simulink model "x20240109_HVDCMMCInterconnection"  (R2023b)
settings: Solver=FixedStepDiscrete  StartTime=0.0  StopTime=2  FixedStep=Ts_Power  RelTol=1e-4  EnableMultiTasking=on
PreLoadFcn:
  | HVDCMMCInterconnectionParam
StartFcn:
  | tic
StopFcn:
  | toc
values from neighbouring files (symbols this model uses):
  C_PM = 1.758e-3    (= 0.001758)    [HVDCMMCInterconnectionParam.m]
  Cg = 50e-9    (= 5e-08)    [HVDCMMCInterconnectionParam.m]
  D_R = 0.001    [HVDCMMCInterconnectionParam.m]
  D_Rs = 1e8    (= 100000000)    [HVDCMMCInterconnectionParam.m]
  D_Vf = 0    [HVDCMMCInterconnectionParam.m]
  Fnom = 50    [HVDCMMCInterconnectionParam.m]
  HRM = 2    [HVDCMMCInterconnectionParam.m]
  Ki_Ireg = 6    [HVDCMMCInterconnectionParam.m]
  Ki_Preg = 1.0    (= 1)    [HVDCMMCInterconnectionParam.m]
  Ki_Qreg = 1.0    (= 1)    [HVDCMMCInterconnectionParam.m]
  Ki_VDCreg = 100    [HVDCMMCInterconnectionParam.m]
  Kp_Ireg = 0.6    [HVDCMMCInterconnectionParam.m]
  Kp_Preg = 0.5/3    (= 0.166666666667)    [HVDCMMCInterconnectionParam.m]
  Kp_Qreg = 0.5/3    (= 0.166666666667)    [HVDCMMCInterconnectionParam.m]
  Kp_VDCreg = 4    [HVDCMMCInterconnectionParam.m]
  L_cable = 15e-3    (= 0.015)    [HVDCMMCInterconnectionParam.m]
  Larm = Larm_pu*(Zb_ac/(2*pi*Fnom))    [HVDCMMCInterconnectionParam.m]
  Lff = Larm_pu/2    (= 0.075)    [HVDCMMCInterconnectionParam.m]
  Limits_Ireg = [ 2.0  -2.0]    [HVDCMMCInterconnectionParam.m]
  Limits_Preg = [ 1.2, 0.8 ]    [HVDCMMCInterconnectionParam.m]
  Limits_Qreg = [ 0.25, -0.25 ]    [HVDCMMCInterconnectionParam.m]
  Limits_VDCreg = [ 2.0  -2.0]    [HVDCMMCInterconnectionParam.m]
  Lxfo = 0.12    [HVDCMMCInterconnectionParam.m]
  Nb_PM = 36    [HVDCMMCInterconnectionParam.m]
  Pnom = 1000e6    (= 1000000000)    [HVDCMMCInterconnectionParam.m]
  R_cable = 0.5    [HVDCMMCInterconnectionParam.m]
  R_startup = 400    [HVDCMMCInterconnectionParam.m]
  Rarm = Rarm_pu*Zb_ac    [HVDCMMCInterconnectionParam.m]
  Rff = Rarm_pu/2    (= 0.00075)    [HVDCMMCInterconnectionParam.m]
  Rg = 100    [HVDCMMCInterconnectionParam.m]
  Rxfo = 0.003    [HVDCMMCInterconnectionParam.m]
  Slope_Pref = 0.5    [HVDCMMCInterconnectionParam.m]
  Slope_Qref = 0.5    [HVDCMMCInterconnectionParam.m]
  Slope_Vdc_ref = Vnom_dc/5    (= 128000)    [HVDCMMCInterconnectionParam.m]
  Tbrk1_On = 0.1    [HVDCMMCInterconnectionParam.m]
  Tbrk2_On = 1.0    (= 1)    [HVDCMMCInterconnectionParam.m]
  Tdeblock = 1.5    [HVDCMMCInterconnectionParam.m]
  Tfault = 9999    [HVDCMMCInterconnectionParam.m]
  Ton_Converter2 = 4    [HVDCMMCInterconnectionParam.m]
  Ton_PQreg = 4    [HVDCMMCInterconnectionParam.m]
  Ton_VDCreg = 1.5    [HVDCMMCInterconnectionParam.m]
  Ts = Ts_Control    (= 4e-05)    [HVDCMMCInterconnectionParam.m]
  Ts_Control = 40e-6    (= 4e-05)    [HVDCMMCInterconnectionParam.m]
  Ts_Power = 20e-6    (= 2e-05)    [HVDCMMCInterconnectionParam.m]
  Vb_ac = sqrt(2/3)*Vnom_sec    [HVDCMMCInterconnectionParam.m]
  Vb_dc = Vnom_dc    (= 640000)    [HVDCMMCInterconnectionParam.m]
  Vc0_PM = 0    [HVDCMMCInterconnectionParam.m]
  Vnom_dc = 640e3    (= 640000)    [HVDCMMCInterconnectionParam.m]
  Vnom_prim = 400e3    (= 400000)    [HVDCMMCInterconnectionParam.m]
  Vnom_sec = 333e3    (= 333000)    [HVDCMMCInterconnectionParam.m]
  w = 2*pi*Fnom    (= 314.159265359)    [HVDCMMCInterconnectionParam.m]
undefined symbols (not defined in the file or in its folder): DiscIntNeverNeededParam, gcbh, Pcc, S, sps_AC, sps_ACDC2, sps_rtmsupport
libraries: simulink x48, spsControlledVoltageSourceLib x30, spsCurrentMeasurementLib x30, MMC_Lib x30, spsDiodeLib x20, spsSeriesRLCBranchLib x14, powerlib_extras x12, spsVoltageMeasurementLib x12, spsSecondOrderFilterLib x8, spsabctodq0Lib x8, spsGroundLib x7, spsMeanLib x4
(part 2 of 9)

== system x20240109_HVDCMMCInterconnection/3ph SM11 ==
  Uref_An : Inport
  An_Ipos : Inport  Port=2
  An_Icap : Inport  Port=3
  Demux : Demux  Outputs=2
  Demux2 : Demux  Outputs=2
  Discrete-Time Integrator1 : DiscreteIntegrator  IntegratorMethod=Integration: Trapezoidal  gainval=1  SampleTime=Ts_Power  UpperSaturationLimit=5000  LowerSaturationLimit=500  ICPrevOutput=DiscIntNeverNeededParam  ICPrevScaledInput=DiscIntNeverNeededParam
  Gain1 : Gain  Gain=Nb_PM
  Gain4 : Gain  Gain=1/(C_PM*Nb_PM)
  Gain5 : Gain  Gain=2
  Mux1 : Mux  Inputs=2
  Mux2 : Mux  Inputs=2
  Product3 : Product
  Product4 : Product
  Product7 : Product
  Sum3 : Sum  Inputs=1  InputSameDT=on  SaturateOnIntegerOverflow=on  OutDataTypeStr=Inherit: Same as first input
  Sum4 : Sum  Inputs=+-  InputSameDT=on  SaturateOnIntegerOverflow=on  OutDataTypeStr=Inherit: Same as first input
  Unit Delay5 : UnitDelay  SampleTime=Ts_Power  HasFrameUpgradeWarning=on
  Unit Delay6 : UnitDelay  SampleTime=Ts_Power  HasFrameUpgradeWarning=on
  Unit Delay7 : UnitDelay  SampleTime=Ts_Power  HasFrameUpgradeWarning=on
  An_Vbl : Outport
  An_Vin : Outport  Port=2
  wires:
  Gain5/1 -> Sum4/1
  Gain1/1 -> Demux2/1, Product3/1
  Mux2/1 -> Demux/1
  Demux/1 -> An_Vin/1
  Uref_An/1 -> Gain1/1
  Gain4/1 -> Discrete-Time Integrator1/1
  Mux1/1 -> Unit Delay7/1
  Demux2/2 -> Product7/1
  Unit Delay6/1 -> Gain5/1, Unit Delay5/1
  An_Icap/1 -> Mux1/2
  Demux2/1 -> Product4/1
  Discrete-Time Integrator1/1 -> Unit Delay6/1
  Sum4/1 -> Product7/2, Product4/2  "Vc"
  Unit Delay5/1 -> Sum4/2
  Sum3/1 -> Gain4/1
  Product3/1 -> Sum3/1
  Product4/1 -> Mux2/1  "Vin"
  Demux/2 -> An_Vbl/1
  Product7/1 -> Mux2/2  "Vbl"
  Unit Delay7/1 -> Product3/2
  An_Ipos/1 -> Mux1/1

== system x20240109_HVDCMMCInterconnection/3ph SM12 ==
  Uref_An : Inport
  An_Ipos : Inport  Port=2
  An_Icap : Inport  Port=3
  Demux : Demux  Outputs=2
  Demux2 : Demux  Outputs=2
  Discrete-Time Integrator1 : DiscreteIntegrator  IntegratorMethod=Integration: Trapezoidal  gainval=1  SampleTime=Ts_Power  UpperSaturationLimit=5000  LowerSaturationLimit=500  ICPrevOutput=DiscIntNeverNeededParam  ICPrevScaledInput=DiscIntNeverNeededParam
  Gain1 : Gain  Gain=Nb_PM
  Gain4 : Gain  Gain=1/(C_PM*Nb_PM)
  Gain5 : Gain  Gain=2
  Mux1 : Mux  Inputs=2
  Mux2 : Mux  Inputs=2
  Product3 : Product
  Product4 : Product
  Product7 : Product
  Sum3 : Sum  Inputs=1  InputSameDT=on  SaturateOnIntegerOverflow=on  OutDataTypeStr=Inherit: Same as first input
  Sum4 : Sum  Inputs=+-  InputSameDT=on  SaturateOnIntegerOverflow=on  OutDataTypeStr=Inherit: Same as first input
  Unit Delay5 : UnitDelay  SampleTime=Ts_Power  HasFrameUpgradeWarning=on
  Unit Delay6 : UnitDelay  SampleTime=Ts_Power  HasFrameUpgradeWarning=on
  Unit Delay7 : UnitDelay  SampleTime=Ts_Power  HasFrameUpgradeWarning=on
  An_Vbl : Outport
  An_Vin : Outport  Port=2
  wires:
  Gain5/1 -> Sum4/1
  Gain1/1 -> Demux2/1, Product3/1
  Mux2/1 -> Demux/1
  Demux/1 -> An_Vin/1
  Uref_An/1 -> Gain1/1
  Gain4/1 -> Discrete-Time Integrator1/1
  Mux1/1 -> Unit Delay7/1
  Demux2/2 -> Product7/1
  Unit Delay6/1 -> Gain5/1, Unit Delay5/1
  An_Icap/1 -> Mux1/2
  Demux2/1 -> Product4/1
  Discrete-Time Integrator1/1 -> Unit Delay6/1
  Sum4/1 -> Product7/2, Product4/2  "Vc"
  Unit Delay5/1 -> Sum4/2
  Sum3/1 -> Gain4/1
  Product3/1 -> Sum3/1
  Product4/1 -> Mux2/1  "Vin"
  Demux/2 -> An_Vbl/1
  Product7/1 -> Mux2/2  "Vbl"
  Unit Delay7/1 -> Product3/2
  An_Ipos/1 -> Mux1/1

== system x20240109_HVDCMMCInterconnection/3ph SM13 ==
  Uref_An : Inport
  An_Ipos : Inport  Port=2
  An_Icap : Inport  Port=3
  Demux : Demux  Outputs=2
  Demux2 : Demux  Outputs=2
  Discrete-Time Integrator1 : DiscreteIntegrator  IntegratorMethod=Integration: Trapezoidal  gainval=1  SampleTime=Ts_Power  UpperSaturationLimit=5000  LowerSaturationLimit=500  ICPrevOutput=DiscIntNeverNeededParam  ICPrevScaledInput=DiscIntNeverNeededParam
  Gain1 : Gain  Gain=Nb_PM
  Gain4 : Gain  Gain=1/(C_PM*Nb_PM)
  Gain5 : Gain  Gain=2
  Mux1 : Mux  Inputs=2
  Mux2 : Mux  Inputs=2
  Product3 : Product
  Product4 : Product
  Product7 : Product
  Sum3 : Sum  Inputs=1  InputSameDT=on  SaturateOnIntegerOverflow=on  OutDataTypeStr=Inherit: Same as first input
  Sum4 : Sum  Inputs=+-  InputSameDT=on  SaturateOnIntegerOverflow=on  OutDataTypeStr=Inherit: Same as first input
  Unit Delay5 : UnitDelay  SampleTime=Ts_Power  HasFrameUpgradeWarning=on
  Unit Delay6 : UnitDelay  SampleTime=Ts_Power  HasFrameUpgradeWarning=on
  Unit Delay7 : UnitDelay  SampleTime=Ts_Power  HasFrameUpgradeWarning=on
  An_Vbl : Outport
  An_Vin : Outport  Port=2
  wires:
  Gain5/1 -> Sum4/1
  Gain1/1 -> Demux2/1, Product3/1
  Mux2/1 -> Demux/1
  Demux/1 -> An_Vin/1
  Uref_An/1 -> Gain1/1
  Gain4/1 -> Discrete-Time Integrator1/1
  Mux1/1 -> Unit Delay7/1
  Demux2/2 -> Product7/1
  Unit Delay6/1 -> Gain5/1, Unit Delay5/1
  An_Icap/1 -> Mux1/2
  Demux2/1 -> Product4/1
  Discrete-Time Integrator1/1 -> Unit Delay6/1
  Sum4/1 -> Product7/2, Product4/2  "Vc"
  Unit Delay5/1 -> Sum4/2
  Sum3/1 -> Gain4/1
  Product3/1 -> Sum3/1
  Product4/1 -> Mux2/1  "Vin"
  Demux/2 -> An_Vbl/1
  Product7/1 -> Mux2/2  "Vbl"
  Unit Delay7/1 -> Product3/2
  An_Ipos/1 -> Mux1/1

== system x20240109_HVDCMMCInterconnection/3ph SM14 ==
  Uref_An : Inport
  An_Ipos : Inport  Port=2
  An_Icap : Inport  Port=3
  Demux : Demux  Outputs=2
  Demux2 : Demux  Outputs=2
  Discrete-Time Integrator1 : DiscreteIntegrator  IntegratorMethod=Integration: Trapezoidal  gainval=1  SampleTime=Ts_Power  UpperSaturationLimit=5000  LowerSaturationLimit=500  ICPrevOutput=DiscIntNeverNeededParam  ICPrevScaledInput=DiscIntNeverNeededParam
  Gain1 : Gain  Gain=Nb_PM
  Gain4 : Gain  Gain=1/(C_PM*Nb_PM)
  Gain5 : Gain  Gain=2
  Mux1 : Mux  Inputs=2
  Mux2 : Mux  Inputs=2
  Product3 : Product
  Product4 : Product
  Product7 : Product
  Sum3 : Sum  Inputs=1  InputSameDT=on  SaturateOnIntegerOverflow=on  OutDataTypeStr=Inherit: Same as first input
  Sum4 : Sum  Inputs=+-  InputSameDT=on  SaturateOnIntegerOverflow=on  OutDataTypeStr=Inherit: Same as first input
  Unit Delay5 : UnitDelay  SampleTime=Ts_Power  HasFrameUpgradeWarning=on
  Unit Delay6 : UnitDelay  SampleTime=Ts_Power  HasFrameUpgradeWarning=on
  Unit Delay7 : UnitDelay  SampleTime=Ts_Power  HasFrameUpgradeWarning=on
  An_Vbl : Outport
  An_Vin : Outport  Port=2
  wires:
  Gain5/1 -> Sum4/1
  Gain1/1 -> Demux2/1, Product3/1
  Mux2/1 -> Demux/1
  Demux/1 -> An_Vin/1
  Uref_An/1 -> Gain1/1
  Gain4/1 -> Discrete-Time Integrator1/1
  Mux1/1 -> Unit Delay7/1
  Demux2/2 -> Product7/1
  Unit Delay6/1 -> Gain5/1, Unit Delay5/1
  An_Icap/1 -> Mux1/2
  Demux2/1 -> Product4/1
  Discrete-Time Integrator1/1 -> Unit Delay6/1
  Sum4/1 -> Product7/2, Product4/2  "Vc"
  Unit Delay5/1 -> Sum4/2
  Sum3/1 -> Gain4/1
  Product3/1 -> Sum3/1
  Product4/1 -> Mux2/1  "Vin"
  Demux/2 -> An_Vbl/1
  Product7/1 -> Mux2/2  "Vbl"
  Unit Delay7/1 -> Product3/2
  An_Ipos/1 -> Mux1/1

== system x20240109_HVDCMMCInterconnection/3ph SM2 ==
  Uref_Ap : Inport
  Ap_Ipos : Inport  Port=2
  Ap_Icap : Inport  Port=3
  Demux1 : Demux  Outputs=2
  Demux3 : Demux  Outputs=2
  Discrete-Time Integrator2 : DiscreteIntegrator  IntegratorMethod=Integration: Trapezoidal  gainval=1  SampleTime=Ts_Power  UpperSaturationLimit=5000  LowerSaturationLimit=500  ICPrevOutput=DiscIntNeverNeededParam  ICPrevScaledInput=DiscIntNeverNeededParam
  Gain2 : Gain  Gain=Nb_PM
  Gain3 : Gain  Gain=1/(C_PM*Nb_PM)
  Gain6 : Gain  Gain=2
  Mux3 : Mux  Inputs=2
  Mux4 : Mux  Inputs=2
  Product1 : Product
  Product2 : Product
  Product5 : Product
  Sum1 : Sum  Inputs=1  InputSameDT=on  SaturateOnIntegerOverflow=on  OutDataTypeStr=Inherit: Same as first input
  Sum2 : Sum  Inputs=+-  InputSameDT=on  SaturateOnIntegerOverflow=on  OutDataTypeStr=Inherit: Same as first input
  Unit Delay1 : UnitDelay  SampleTime=Ts_Power  HasFrameUpgradeWarning=on
  Unit Delay2 : UnitDelay  SampleTime=Ts_Power  HasFrameUpgradeWarning=on
  Unit Delay3 : UnitDelay  SampleTime=Ts_Power  HasFrameUpgradeWarning=on
  Ap_Vbl : Outport
  Ap_Vin : Outport  Port=2
  wires:
  Demux1/2 -> Ap_Vbl/1
  Ap_Ipos/1 -> Mux3/1
  Unit Delay3/1 -> Product1/2
  Product1/1 -> Sum1/1
  Sum1/1 -> Gain3/1
  Unit Delay1/1 -> Sum2/2
  Sum2/1 -> Product5/2, Product2/2  "Vc"
  Uref_Ap/1 -> Gain2/1
  Unit Delay2/1 -> Gain6/1, Unit Delay1/1
  Mux3/1 -> Unit Delay3/1
  Demux3/2 -> Product5/1
  Gain3/1 -> Discrete-Time Integrator2/1
  Gain2/1 -> Demux3/1, Product1/1
  Demux3/1 -> Product2/1
  Demux1/1 -> Ap_Vin/1
  Mux4/1 -> Demux1/1
  Product2/1 -> Mux4/1  "Vin"
  Discrete-Time Integrator2/1 -> Unit Delay2/1
  Ap_Icap/1 -> Mux3/2
  Gain6/1 -> Sum2/1
  Product5/1 -> Mux4/2  "Vbl"

== system x20240109_HVDCMMCInterconnection/3ph SM9 ==
  Uref_An : Inport
  An_Ipos : Inport  Port=2
  An_Icap : Inport  Port=3
  Demux : Demux  Outputs=2
  Demux2 : Demux  Outputs=2
  Discrete-Time Integrator1 : DiscreteIntegrator  IntegratorMethod=Integration: Trapezoidal  gainval=1  SampleTime=Ts_Power  UpperSaturationLimit=5000  LowerSaturationLimit=500  ICPrevOutput=DiscIntNeverNeededParam  ICPrevScaledInput=DiscIntNeverNeededParam
  Gain1 : Gain  Gain=Nb_PM
  Gain4 : Gain  Gain=1/(C_PM*Nb_PM)
  Gain5 : Gain  Gain=2
  Mux1 : Mux  Inputs=2
  Mux2 : Mux  Inputs=2
  Product3 : Product
  Product4 : Product
  Product7 : Product
  Sum3 : Sum  Inputs=1  InputSameDT=on  SaturateOnIntegerOverflow=on  OutDataTypeStr=Inherit: Same as first input
  Sum4 : Sum  Inputs=+-  InputSameDT=on  SaturateOnIntegerOverflow=on  OutDataTypeStr=Inherit: Same as first input
  Unit Delay5 : UnitDelay  SampleTime=Ts_Power  HasFrameUpgradeWarning=on
  Unit Delay6 : UnitDelay  SampleTime=Ts_Power  HasFrameUpgradeWarning=on
  Unit Delay7 : UnitDelay  SampleTime=Ts_Power  HasFrameUpgradeWarning=on
  An_Vbl : Outport
  An_Vin : Outport  Port=2
  wires:
  Gain5/1 -> Sum4/1
  Gain1/1 -> Demux2/1, Product3/1
  Mux2/1 -> Demux/1
  Demux/1 -> An_Vin/1
  Uref_An/1 -> Gain1/1
  Gain4/1 -> Discrete-Time Integrator1/1
  Mux1/1 -> Unit Delay7/1
  Demux2/2 -> Product7/1
  Unit Delay6/1 -> Gain5/1, Unit Delay5/1
  An_Icap/1 -> Mux1/2
  Demux2/1 -> Product4/1
  Discrete-Time Integrator1/1 -> Unit Delay6/1
  Sum4/1 -> Product7/2, Product4/2  "Vc"
  Unit Delay5/1 -> Sum4/2
  Sum3/1 -> Gain4/1
  Product3/1 -> Sum3/1
  Product4/1 -> Mux2/1  "Vin"
  Demux/2 -> An_Vbl/1
  Product7/1 -> Mux2/2  "Vbl"
  Unit Delay7/1 -> Product3/2
  An_Ipos/1 -> Mux1/1

== system x20240109_HVDCMMCInterconnection/Control ==
  PQreg_ON : Inport
  Vdc_ref : Inport  Port=2
  Qref : Inport  Port=3
  Vsec : Inport  Port=4
  Isec : Inport  Port=5
  Active Power Regulator (Preg) : Subsystem
  Bus Creator : BusCreator  Inputs=8
  Current Regulator (Ireg) : Subsystem
      settings: PortSchema="{\"entries\":[{\"content\":{\"sides\":[{\"content\":{\"connectorIds\":[\"In1\",\"In2\",\"In3\",\"In4\",\"In5\"]},\"type\":\"ConnectorPlacement.EquallySpacedRectSide\",\"uuid\":\"46fff04e-1450-479d-b460-437d90e99f23\"},{\"content\":{\"connectorIds\":[\"Out1\",\"Out2\",\"Out3\"],\"side\":\"RIGHT\"},\"type\":\"ConnectorPlacement.EquallySpacedRectSide\",\"uuid\":\"1fecc714-62d0-4152-98c9-212d930a5fef\"},{\"content\":{\"connectorIds\":[\"In6\"],\"side\":\"TOP\"},\"type\":\"ConnectorPlacement.EquallySpacedRectSide\",\"uuid\":\"861e6320-ec6e-4c2a-8449-e621a478dd1e\"}]},\"type\":\"ConnectorPlacement.EquallySpacedConnector\",\"uuid\":\"2e901dc7-e129-44fe-b6c0-1fa97996cfbd\"}],\"packageUris\":[\"http://schema.mathworks.com/mf0/Connector/R2020b\"],\"version\":\"1.0\"}"
  DC Voltage Regulator (VDCreg) : Subsystem
      settings: PortSchema="{\"entries\":[{\"content\":{\"sides\":[{\"content\":{\"connectorIds\":[\"In1\",\"In2\"]},\"type\":\"ConnectorPlacement.EquallySpacedRectSide\",\"uuid\":\"c20f24de-2933-46ae-a608-0dc6cbdc22c5\"},{\"content\":{\"connectorIds\":[\"Out1\"],\"side\":\"RIGHT\"},\"type\":\"ConnectorPlacement.EquallySpacedRectSide\",\"uuid\":\"78958689-3494-4241-b4e6-c71b7d261298\"},{\"content\":{\"connectorIds\":[\"In3\"],\"side\":\"TOP\"},\"type\":\"ConnectorPlacement.EquallySpacedRectSide\",\"uuid\":\"05cc66e2-c7d6-407f-b011-a28bc71811d6\"}]},\"type\":\"ConnectorPlacement.EquallySpacedConnector\",\"uuid\":\"0d848e7c-ac8e-4664-bac3-455723337427\"}],\"packageUris\":[\"http://schema.mathworks.com/mf0/Connector/R2020b\"],\"version\":\"1.0\"}"
  Demux1 : Demux  Outputs=2
  Demux3 : Demux  Outputs=2
  Mux : Mux  Inputs=2
  Mux1 : Mux  Inputs=2
  Mux2 : Mux  Inputs=2
  "PLL, Measurements and Transformation" : Subsystem
      settings: PortSchema="{\"entries\":[{\"content\":{\"sides\":[{\"content\":{\"connectorIds\":[\"In1\",\"In2\"]},\"type\":\"ConnectorPlacement.EquallySpacedRectSide\",\"uuid\":\"b10cca13-b0c2-430a-b17c-db71eb4f1a3c\"},{\"content\":{\"connectorIds\":[\"Out1\",\"Out2\",\"Out3\",\"Out4\"],\"side\":\"RIGHT\"},\"type\":\"ConnectorPlacement.EquallySpacedRectSide\",\"uuid\":\"355382eb-bc30-4f3c-94e5-48c8b9c2ecfd\"},{\"content\":{\"connectorIds\":[\"Out5\",\"Out6\"],\"side\":\"TOP\"},\"type\":\"ConnectorPlacement.EquallySpacedRectSide\",\"uuid\":\"77f94122-ff4d-41eb-b55d-9b38525f3ab4\"}]},\"type\":\"ConnectorPlacement.EquallySpacedConnector\",\"uuid\":\"46538cda-22c7-46a2-9cc9-63f6dc7214f2\"}],\"packageUris\":[\"http://schema.mathworks.com/mf0/Connector/R2020b\"],\"version\":\"1.0\"}"
  Rate Transition{,1..2,7} (4 alike) : RateTransition  OutPortSampleTime=Ts_Control
  Rate Transition11 : RateTransition  OutPortSampleTime=Ts_Power
  Rate Transition3 : RateTransition  OutPortSampleTime=Ts_Power
  Rate Transition4 : RateTransition  OutPortSampleTime=Ts_Power
  Reactive Power Regulator : Subsystem
      settings: PortSchema="{\"entries\":[{\"content\":{\"sides\":[{\"content\":{\"connectorIds\":[\"In1\",\"In2\"]},\"type\":\"ConnectorPlacement.EquallySpacedRectSide\",\"uuid\":\"eeeb811d-908b-486e-b0fa-0b5fd0d6695a\"},{\"content\":{\"connectorIds\":[\"Out1\"],\"side\":\"RIGHT\"},\"type\":\"ConnectorPlacement.EquallySpacedRectSide\",\"uuid\":\"28c9bf02-c5ab-433a-87a9-c17e67d0c029\"},{\"content\":{\"side\":\"TOP\"},\"type\":\"ConnectorPlacement.EquallySpacedRectSide\",\"uuid\":\"fdca837a-4079-4910-a6d7-edbb284eaa51\"},{\"content\":{\"connectorIds\":[\"In3\",\"In4\"],\"side\":\"BOTTOM\"},\"type\":\"ConnectorPlacement.EquallySpacedRectSide\",\"uuid\":\"d2fa5805-110b-4a78-bf6e-301fd334a724\"}]},\"type\":\"ConnectorPlacement.EquallySpacedConnector\",\"uuid\":\"cbc8ea8f-55f5-4ff6-b34f-d5812b415dcf\"}],\"packageUris\":[\"http://schema.mathworks.com/mf0/Connector/R2020b\"],\"version\":\"1.0\"}"
  Switch : Switch  Criteria=u2 ~= 0  SaturateOnIntegerOverflow=off  InputSameDT=off
  Uref : Outport
  Meas : Outport  Port=2
  m1_dq : Outport  Port=3
  wt : Outport  Port=4
  wires:
  Mux1/1 -> Bus Creator/7  "PrefPmeas"
  "PLL, Measurements and Transformation"/4(P) -> Mux1/2, Active Power Regulator (Preg)/1(Pmeas)
  DC Voltage Regulator (VDCreg)/1(Id_ref) -> Mux/1
  "PLL, Measurements and Transformation"/2(wt) -> Rate Transition4/1, Current Regulator (Ireg)/4(wt)
  Demux1/1 -> Bus Creator/3  "Id"
  Vsec/1 -> Rate Transition1/1
  "PLL, Measurements and Transformation"/6(VdVq) -> Reactive Power Regulator/4(VdVq_mes), Current Regulator (Ireg)/2(VdVq)
  Mux2/1 -> [QrefQmeas]
  Rate Transition11/1 -> Uref/1
  "PLL, Measurements and Transformation"/5(Q) -> Mux2/2, Reactive Power Regulator/3(Qmes)
  [Pref] -> Active Power Regulator (Preg)/2(Pref), Mux1/1
  Isec/1 -> Rate Transition2/1
  [PQreg_On] -> Active Power Regulator (Preg)/3(On)
  [QrefQmeas] -> Bus Creator/8  "QrefQmeas"
  Current Regulator (Ireg)/2(m) -> Rate Transition3/1, Rate Transition7/1
  Demux3/2 -> Bus Creator/2  "Iqref"
  Rate Transition7/1 -> Bus Creator/5  "m"
  [Vdc_ref_Preg] -> Switch/1
  Demux3/1 -> Bus Creator/1  "Idref"
  Mux/1 -> Demux3/1, Current Regulator (Ireg)/1(IdIq_ref)
  Switch/1 -> DC Voltage Regulator (VDCreg)/1(Vdc_ref)
  Current Regulator (Ireg)/3(PIdq) -> Bus Creator/6  "PIdq"
  [Vdc1] -> Rate Transition/1
  PQreg_ON/1 -> Reactive Power Regulator/1(On), Switch/2
  Rate Transition1/1 -> "PLL, Measurements and Transformation"/1(Vabc)
  "PLL, Measurements and Transformation"/1(Freq) -> Current Regulator (Ireg)/3(Freq)
  Vdc_ref/1 -> Switch/3
  Active Power Regulator (Preg)/1(Vdc_ref) -> [Vdc_ref_Preg]
  Rate Transition2/1 -> "PLL, Measurements and Transformation"/2(Iabc)
  Rate Transition/1 -> DC Voltage Regulator (VDCreg)/3(Vdc_meas), Current Regulator (Ireg)/6(Vdc)
  [VDCreg_On] -> DC Voltage Regulator (VDCreg)/2(On)
  Demux1/2 -> Bus Creator/4  "Iq"
  "PLL, Measurements and Transformation"/3(IdIq) -> Current Regulator (Ireg)/5(IdIq), Demux1/1
  Qref/1 -> Mux2/1, Reactive Power Regulator/2(Qref)
  Current Regulator (Ireg)/1(Uref_ABC) -> Rate Transition11/1
  Bus Creator/1 -> Meas/1
  Reactive Power Regulator/1(Iq_ref) -> Mux/2
  Rate Transition3/1 -> m1_dq/1
  Rate Transition4/1 -> wt/1

== system x20240109_HVDCMMCInterconnection/Control1 ==
  PQreg_ON : Inport
  Vdc_ref : Inport  Port=2
  Qref : Inport  Port=3
  Vsec : Inport  Port=4
  Isec : Inport  Port=5
  Active Power Regulator (Preg) : Subsystem
  Bus Creator : BusCreator  Inputs=8
  Current Regulator (Ireg) : Subsystem
      settings: PortSchema="{\"entries\":[{\"content\":{\"sides\":[{\"content\":{\"connectorIds\":[\"In1\",\"In2\",\"In3\",\"In4\",\"In5\"]},\"type\":\"ConnectorPlacement.EquallySpacedRectSide\",\"uuid\":\"46fff04e-1450-479d-b460-437d90e99f23\"},{\"content\":{\"connectorIds\":[\"Out1\",\"Out2\",\"Out3\"],\"side\":\"RIGHT\"},\"type\":\"ConnectorPlacement.EquallySpacedRectSide\",\"uuid\":\"1fecc714-62d0-4152-98c9-212d930a5fef\"},{\"content\":{\"connectorIds\":[\"In6\"],\"side\":\"TOP\"},\"type\":\"ConnectorPlacement.EquallySpacedRectSide\",\"uuid\":\"861e6320-ec6e-4c2a-8449-e621a478dd1e\"}]},\"type\":\"ConnectorPlacement.EquallySpacedConnector\",\"uuid\":\"2e901dc7-e129-44fe-b6c0-1fa97996cfbd\"}],\"packageUris\":[\"http://schema.mathworks.com/mf0/Connector/R2020b\"],\"version\":\"1.0\"}"
  DC Voltage Regulator (VDCreg) : Subsystem
      settings: PortSchema="{\"entries\":[{\"content\":{\"sides\":[{\"content\":{\"connectorIds\":[\"In1\",\"In2\"]},\"type\":\"ConnectorPlacement.EquallySpacedRectSide\",\"uuid\":\"c20f24de-2933-46ae-a608-0dc6cbdc22c5\"},{\"content\":{\"connectorIds\":[\"Out1\"],\"side\":\"RIGHT\"},\"type\":\"ConnectorPlacement.EquallySpacedRectSide\",\"uuid\":\"78958689-3494-4241-b4e6-c71b7d261298\"},{\"content\":{\"connectorIds\":[\"In3\"],\"side\":\"TOP\"},\"type\":\"ConnectorPlacement.EquallySpacedRectSide\",\"uuid\":\"05cc66e2-c7d6-407f-b011-a28bc71811d6\"}]},\"type\":\"ConnectorPlacement.EquallySpacedConnector\",\"uuid\":\"0d848e7c-ac8e-4664-bac3-455723337427\"}],\"packageUris\":[\"http://schema.mathworks.com/mf0/Connector/R2020b\"],\"version\":\"1.0\"}"
  Demux1 : Demux  Outputs=2
  Demux3 : Demux  Outputs=2
  Mux : Mux  Inputs=2
  Mux1 : Mux  Inputs=2
  Mux2 : Mux  Inputs=2
  "PLL, Measurements and Transformation" : Subsystem
      settings: PortSchema="{\"entries\":[{\"content\":{\"sides\":[{\"content\":{\"connectorIds\":[\"In1\",\"In2\"]},\"type\":\"ConnectorPlacement.EquallySpacedRectSide\",\"uuid\":\"b10cca13-b0c2-430a-b17c-db71eb4f1a3c\"},{\"content\":{\"connectorIds\":[\"Out1\",\"Out2\",\"Out3\",\"Out4\"],\"side\":\"RIGHT\"},\"type\":\"ConnectorPlacement.EquallySpacedRectSide\",\"uuid\":\"355382eb-bc30-4f3c-94e5-48c8b9c2ecfd\"},{\"content\":{\"connectorIds\":[\"Out5\",\"Out6\"],\"side\":\"TOP\"},\"type\":\"ConnectorPlacement.EquallySpacedRectSide\",\"uuid\":\"77f94122-ff4d-41eb-b55d-9b38525f3ab4\"}]},\"type\":\"ConnectorPlacement.EquallySpacedConnector\",\"uuid\":\"46538cda-22c7-46a2-9cc9-63f6dc7214f2\"}],\"packageUris\":[\"http://schema.mathworks.com/mf0/Connector/R2020b\"],\"version\":\"1.0\"}"
  Rate Transition{,1..2,7} (4 alike) : RateTransition  OutPortSampleTime=Ts_Control
  Rate Transition11 : RateTransition  OutPortSampleTime=Ts_Power
  Rate Transition3 : RateTransition  OutPortSampleTime=Ts_Power
  Rate Transition4 : RateTransition  OutPortSampleTime=Ts_Power
  Reactive Power Regulator : Subsystem
      settings: PortSchema="{\"entries\":[{\"content\":{\"sides\":[{\"content\":{\"connectorIds\":[\"In1\",\"In2\"]},\"type\":\"ConnectorPlacement.EquallySpacedRectSide\",\"uuid\":\"eeeb811d-908b-486e-b0fa-0b5fd0d6695a\"},{\"content\":{\"connectorIds\":[\"Out1\"],\"side\":\"RIGHT\"},\"type\":\"ConnectorPlacement.EquallySpacedRectSide\",\"uuid\":\"28c9bf02-c5ab-433a-87a9-c17e67d0c029\"},{\"content\":{\"side\":\"TOP\"},\"type\":\"ConnectorPlacement.EquallySpacedRectSide\",\"uuid\":\"fdca837a-4079-4910-a6d7-edbb284eaa51\"},{\"content\":{\"connectorIds\":[\"In3\",\"In4\"],\"side\":\"BOTTOM\"},\"type\":\"ConnectorPlacement.EquallySpacedRectSide\",\"uuid\":\"d2fa5805-110b-4a78-bf6e-301fd334a724\"}]},\"type\":\"ConnectorPlacement.EquallySpacedConnector\",\"uuid\":\"cbc8ea8f-55f5-4ff6-b34f-d5812b415dcf\"}],\"packageUris\":[\"http://schema.mathworks.com/mf0/Connector/R2020b\"],\"version\":\"1.0\"}"
  Switch : Switch  Criteria=u2 ~= 0  SaturateOnIntegerOverflow=off  InputSameDT=off
  Uref : Outport
  Meas : Outport  Port=2
  m1_dq : Outport  Port=3
  wt : Outport  Port=4
  wires:
  Mux1/1 -> Bus Creator/7  "PrefPmeas"
  "PLL, Measurements and Transformation"/4(P) -> Mux1/2, Active Power Regulator (Preg)/1(Pmeas)
  DC Voltage Regulator (VDCreg)/1(Id_ref) -> Mux/1
  "PLL, Measurements and Transformation"/2(wt) -> Rate Transition4/1, Current Regulator (Ireg)/4(wt)
  Demux1/1 -> Bus Creator/3  "Id"
  Vsec/1 -> Rate Transition1/1
  "PLL, Measurements and Transformation"/6(VdVq) -> Reactive Power Regulator/4(VdVq_mes), Current Regulator (Ireg)/2(VdVq)
  Mux2/1 -> [QrefQmeas]
  Rate Transition11/1 -> Uref/1
  "PLL, Measurements and Transformation"/5(Q) -> Mux2/2, Reactive Power Regulator/3(Qmes)
  [Pref] -> Active Power Regulator (Preg)/2(Pref), Mux1/1
  Isec/1 -> Rate Transition2/1
  [PQreg_On] -> Active Power Regulator (Preg)/3(On)
  [QrefQmeas] -> Bus Creator/8  "QrefQmeas"
  Current Regulator (Ireg)/2(m) -> Rate Transition3/1, Rate Transition7/1
  Demux3/2 -> Bus Creator/2  "Iqref"
  Rate Transition7/1 -> Bus Creator/5  "m"
  [Vdc_ref_Preg] -> Switch/1
  Demux3/1 -> Bus Creator/1  "Idref"
  Mux/1 -> Demux3/1, Current Regulator (Ireg)/1(IdIq_ref)
  Switch/1 -> DC Voltage Regulator (VDCreg)/1(Vdc_ref)
  Current Regulator (Ireg)/3(PIdq) -> Bus Creator/6  "PIdq"
  [Vdc1] -> Rate Transition/1
  PQreg_ON/1 -> Reactive Power Regulator/1(On), Switch/2
  Rate Transition1/1 -> "PLL, Measurements and Transformation"/1(Vabc)
  "PLL, Measurements and Transformation"/1(Freq) -> Current Regulator (Ireg)/3(Freq)
  Vdc_ref/1 -> Switch/3
  Active Power Regulator (Preg)/1(Vdc_ref) -> [Vdc_ref_Preg]
  Rate Transition2/1 -> "PLL, Measurements and Transformation"/2(Iabc)
  Rate Transition/1 -> DC Voltage Regulator (VDCreg)/3(Vdc_meas), Current Regulator (Ireg)/6(Vdc)
  [VDCreg_On] -> DC Voltage Regulator (VDCreg)/2(On)
  Demux1/2 -> Bus Creator/4  "Iq"
  "PLL, Measurements and Transformation"/3(IdIq) -> Current Regulator (Ireg)/5(IdIq), Demux1/1
  Qref/1 -> Mux2/1, Reactive Power Regulator/2(Qref)
  Current Regulator (Ireg)/1(Uref_ABC) -> Rate Transition11/1
  Bus Creator/1 -> Meas/1
  Reactive Power Regulator/1(Iq_ref) -> Mux/2
  Rate Transition3/1 -> m1_dq/1
  Rate Transition4/1 -> wt/1

== system x20240109_HVDCMMCInterconnection/Control2 ==
  PQreg_ON : Inport
  Vdc_ref : Inport  Port=2
  Qref : Inport  Port=3
  Vsec : Inport  Port=4
  Isec : Inport  Port=5
  Active Power Regulator (Preg) : Subsystem
  Bus Creator : BusCreator  Inputs=8
  Current Regulator (Ireg) : Subsystem
      settings: PortSchema="{\"entries\":[{\"content\":{\"sides\":[{\"content\":{\"connectorIds\":[\"In1\",\"In2\",\"In3\",\"In4\",\"In5\"]},\"type\":\"ConnectorPlacement.EquallySpacedRectSide\",\"uuid\":\"46fff04e-1450-479d-b460-437d90e99f23\"},{\"content\":{\"connectorIds\":[\"Out1\",\"Out2\",\"Out3\"],\"side\":\"RIGHT\"},\"type\":\"ConnectorPlacement.EquallySpacedRectSide\",\"uuid\":\"1fecc714-62d0-4152-98c9-212d930a5fef\"},{\"content\":{\"connectorIds\":[\"In6\"],\"side\":\"TOP\"},\"type\":\"ConnectorPlacement.EquallySpacedRectSide\",\"uuid\":\"861e6320-ec6e-4c2a-8449-e621a478dd1e\"}]},\"type\":\"ConnectorPlacement.EquallySpacedConnector\",\"uuid\":\"2e901dc7-e129-44fe-b6c0-1fa97996cfbd\"}],\"packageUris\":[\"http://schema.mathworks.com/mf0/Connector/R2020b\"],\"version\":\"1.0\"}"
  DC Voltage Regulator (VDCreg) : Subsystem
      settings: PortSchema="{\"entries\":[{\"content\":{\"sides\":[{\"content\":{\"connectorIds\":[\"In1\",\"In2\"]},\"type\":\"ConnectorPlacement.EquallySpacedRectSide\",\"uuid\":\"c20f24de-2933-46ae-a608-0dc6cbdc22c5\"},{\"content\":{\"connectorIds\":[\"Out1\"],\"side\":\"RIGHT\"},\"type\":\"ConnectorPlacement.EquallySpacedRectSide\",\"uuid\":\"78958689-3494-4241-b4e6-c71b7d261298\"},{\"content\":{\"connectorIds\":[\"In3\"],\"side\":\"TOP\"},\"type\":\"ConnectorPlacement.EquallySpacedRectSide\",\"uuid\":\"05cc66e2-c7d6-407f-b011-a28bc71811d6\"}]},\"type\":\"ConnectorPlacement.EquallySpacedConnector\",\"uuid\":\"0d848e7c-ac8e-4664-bac3-455723337427\"}],\"packageUris\":[\"http://schema.mathworks.com/mf0/Connector/R2020b\"],\"version\":\"1.0\"}"
  Demux1 : Demux  Outputs=2
  Demux3 : Demux  Outputs=2
  Mux : Mux  Inputs=2
  Mux1 : Mux  Inputs=2
  Mux2 : Mux  Inputs=2
  "PLL, Measurements and Transformation" : Subsystem
      settings: PortSchema="{\"entries\":[{\"content\":{\"sides\":[{\"content\":{\"connectorIds\":[\"In1\",\"In2\"]},\"type\":\"ConnectorPlacement.EquallySpacedRectSide\",\"uuid\":\"b10cca13-b0c2-430a-b17c-db71eb4f1a3c\"},{\"content\":{\"connectorIds\":[\"Out1\",\"Out2\",\"Out3\",\"Out4\"],\"side\":\"RIGHT\"},\"type\":\"ConnectorPlacement.EquallySpacedRectSide\",\"uuid\":\"355382eb-bc30-4f3c-94e5-48c8b9c2ecfd\"},{\"content\":{\"connectorIds\":[\"Out5\",\"Out6\"],\"side\":\"TOP\"},\"type\":\"ConnectorPlacement.EquallySpacedRectSide\",\"uuid\":\"77f94122-ff4d-41eb-b55d-9b38525f3ab4\"}]},\"type\":\"ConnectorPlacement.EquallySpacedConnector\",\"uuid\":\"46538cda-22c7-46a2-9cc9-63f6dc7214f2\"}],\"packageUris\":[\"http://schema.mathworks.com/mf0/Connector/R2020b\"],\"version\":\"1.0\"}"
  Rate Transition{,1..2,7} (4 alike) : RateTransition  OutPortSampleTime=Ts_Control
  Rate Transition11 : RateTransition  OutPortSampleTime=Ts_Power
  Rate Transition3 : RateTransition  OutPortSampleTime=Ts_Power
  Rate Transition4 : RateTransition  OutPortSampleTime=Ts_Power
  Reactive Power Regulator : Subsystem
      settings: PortSchema="{\"entries\":[{\"content\":{\"sides\":[{\"content\":{\"connectorIds\":[\"In1\",\"In2\"]},\"type\":\"ConnectorPlacement.EquallySpacedRectSide\",\"uuid\":\"eeeb811d-908b-486e-b0fa-0b5fd0d6695a\"},{\"content\":{\"connectorIds\":[\"Out1\"],\"side\":\"RIGHT\"},\"type\":\"ConnectorPlacement.EquallySpacedRectSide\",\"uuid\":\"28c9bf02-c5ab-433a-87a9-c17e67d0c029\"},{\"content\":{\"side\":\"TOP\"},\"type\":\"ConnectorPlacement.EquallySpacedRectSide\",\"uuid\":\"fdca837a-4079-4910-a6d7-edbb284eaa51\"},{\"content\":{\"connectorIds\":[\"In3\",\"In4\"],\"side\":\"BOTTOM\"},\"type\":\"ConnectorPlacement.EquallySpacedRectSide\",\"uuid\":\"d2fa5805-110b-4a78-bf6e-301fd334a724\"}]},\"type\":\"ConnectorPlacement.EquallySpacedConnector\",\"uuid\":\"cbc8ea8f-55f5-4ff6-b34f-d5812b415dcf\"}],\"packageUris\":[\"http://schema.mathworks.com/mf0/Connector/R2020b\"],\"version\":\"1.0\"}"
  Switch : Switch  Criteria=u2 ~= 0  SaturateOnIntegerOverflow=off  InputSameDT=off
  Uref : Outport
  Meas : Outport  Port=2
  m1_dq : Outport  Port=3
  wt : Outport  Port=4
  wires:
  Mux1/1 -> Bus Creator/7  "PrefPmeas"
  "PLL, Measurements and Transformation"/4(P) -> Mux1/2, Active Power Regulator (Preg)/1(Pmeas)
  DC Voltage Regulator (VDCreg)/1(Id_ref) -> Mux/1
  "PLL, Measurements and Transformation"/2(wt) -> Rate Transition4/1, Current Regulator (Ireg)/4(wt)
  Demux1/1 -> Bus Creator/3  "Id"
  Vsec/1 -> Rate Transition1/1
  "PLL, Measurements and Transformation"/6(VdVq) -> Reactive Power Regulator/4(VdVq_mes), Current Regulator (Ireg)/2(VdVq)
  Mux2/1 -> [QrefQmeas]
  Rate Transition11/1 -> Uref/1
  "PLL, Measurements and Transformation"/5(Q) -> Mux2/2, Reactive Power Regulator/3(Qmes)
  [Pref] -> Active Power Regulator (Preg)/2(Pref), Mux1/1
  Isec/1 -> Rate Transition2/1
  [PQreg_On] -> Active Power Regulator (Preg)/3(On)
  [QrefQmeas] -> Bus Creator/8  "QrefQmeas"
  Current Regulator (Ireg)/2(m) -> Rate Transition3/1, Rate Transition7/1
  Demux3/2 -> Bus Creator/2  "Iqref"
  Rate Transition7/1 -> Bus Creator/5  "m"
  [Vdc_ref_Preg] -> Switch/1
  Demux3/1 -> Bus Creator/1  "Idref"
  Mux/1 -> Demux3/1, Current Regulator (Ireg)/1(IdIq_ref)
  Switch/1 -> DC Voltage Regulator (VDCreg)/1(Vdc_ref)
  Current Regulator (Ireg)/3(PIdq) -> Bus Creator/6  "PIdq"
  [Vdc1] -> Rate Transition/1
  PQreg_ON/1 -> Reactive Power Regulator/1(On), Switch/2
  Rate Transition1/1 -> "PLL, Measurements and Transformation"/1(Vabc)
  "PLL, Measurements and Transformation"/1(Freq) -> Current Regulator (Ireg)/3(Freq)
  Vdc_ref/1 -> Switch/3
  Active Power Regulator (Preg)/1(Vdc_ref) -> [Vdc_ref_Preg]
  Rate Transition2/1 -> "PLL, Measurements and Transformation"/2(Iabc)
  Rate Transition/1 -> DC Voltage Regulator (VDCreg)/3(Vdc_meas), Current Regulator (Ireg)/6(Vdc)
  [VDCreg_On] -> DC Voltage Regulator (VDCreg)/2(On)
  Demux1/2 -> Bus Creator/4  "Iq"
  "PLL, Measurements and Transformation"/3(IdIq) -> Current Regulator (Ireg)/5(IdIq), Demux1/1
  Qref/1 -> Mux2/1, Reactive Power Regulator/2(Qref)
  Current Regulator (Ireg)/1(Uref_ABC) -> Rate Transition11/1
  Bus Creator/1 -> Meas/1
  Reactive Power Regulator/1(Iq_ref) -> Mux/2
  Rate Transition3/1 -> m1_dq/1
  Rate Transition4/1 -> wt/1

== system x20240109_HVDCMMCInterconnection/Control3 ==
  PQreg_ON : Inport
  Vdc_ref : Inport  Port=2
  Qref : Inport  Port=3
  Vsec : Inport  Port=4
  Isec : Inport  Port=5
  Active Power Regulator (Preg) : Subsystem
  Bus Creator : BusCreator  Inputs=8
  Current Regulator (Ireg) : Subsystem
      settings: PortSchema="{\"entries\":[{\"content\":{\"sides\":[{\"content\":{\"connectorIds\":[\"In1\",\"In2\",\"In3\",\"In4\",\"In5\"]},\"type\":\"ConnectorPlacement.EquallySpacedRectSide\",\"uuid\":\"46fff04e-1450-479d-b460-437d90e99f23\"},{\"content\":{\"connectorIds\":[\"Out1\",\"Out2\",\"Out3\"],\"side\":\"RIGHT\"},\"type\":\"ConnectorPlacement.EquallySpacedRectSide\",\"uuid\":\"1fecc714-62d0-4152-98c9-212d930a5fef\"},{\"content\":{\"connectorIds\":[\"In6\"],\"side\":\"TOP\"},\"type\":\"ConnectorPlacement.EquallySpacedRectSide\",\"uuid\":\"861e6320-ec6e-4c2a-8449-e621a478dd1e\"}]},\"type\":\"ConnectorPlacement.EquallySpacedConnector\",\"uuid\":\"2e901dc7-e129-44fe-b6c0-1fa97996cfbd\"}],\"packageUris\":[\"http://schema.mathworks.com/mf0/Connector/R2020b\"],\"version\":\"1.0\"}"
  DC Voltage Regulator (VDCreg) : Subsystem
      settings: PortSchema="{\"entries\":[{\"content\":{\"sides\":[{\"content\":{\"connectorIds\":[\"In1\",\"In2\"]},\"type\":\"ConnectorPlacement.EquallySpacedRectSide\",\"uuid\":\"c20f24de-2933-46ae-a608-0dc6cbdc22c5\"},{\"content\":{\"connectorIds\":[\"Out1\"],\"side\":\"RIGHT\"},\"type\":\"ConnectorPlacement.EquallySpacedRectSide\",\"uuid\":\"78958689-3494-4241-b4e6-c71b7d261298\"},{\"content\":{\"connectorIds\":[\"In3\"],\"side\":\"TOP\"},\"type\":\"ConnectorPlacement.EquallySpacedRectSide\",\"uuid\":\"05cc66e2-c7d6-407f-b011-a28bc71811d6\"}]},\"type\":\"ConnectorPlacement.EquallySpacedConnector\",\"uuid\":\"0d848e7c-ac8e-4664-bac3-455723337427\"}],\"packageUris\":[\"http://schema.mathworks.com/mf0/Connector/R2020b\"],\"version\":\"1.0\"}"
  Demux1 : Demux  Outputs=2
  Demux3 : Demux  Outputs=2
  Mux : Mux  Inputs=2
  Mux1 : Mux  Inputs=2
  Mux2 : Mux  Inputs=2
  "PLL, Measurements and Transformation" : Subsystem
      settings: PortSchema="{\"entries\":[{\"content\":{\"sides\":[{\"content\":{\"connectorIds\":[\"In1\",\"In2\"]},\"type\":\"ConnectorPlacement.EquallySpacedRectSide\",\"uuid\":\"b10cca13-b0c2-430a-b17c-db71eb4f1a3c\"},{\"content\":{\"connectorIds\":[\"Out1\",\"Out2\",\"Out3\",\"Out4\"],\"side\":\"RIGHT\"},\"type\":\"ConnectorPlacement.EquallySpacedRectSide\",\"uuid\":\"355382eb-bc30-4f3c-94e5-48c8b9c2ecfd\"},{\"content\":{\"connectorIds\":[\"Out5\",\"Out6\"],\"side\":\"TOP\"},\"type\":\"ConnectorPlacement.EquallySpacedRectSide\",\"uuid\":\"77f94122-ff4d-41eb-b55d-9b38525f3ab4\"}]},\"type\":\"ConnectorPlacement.EquallySpacedConnector\",\"uuid\":\"46538cda-22c7-46a2-9cc9-63f6dc7214f2\"}],\"packageUris\":[\"http://schema.mathworks.com/mf0/Connector/R2020b\"],\"version\":\"1.0\"}"
  Rate Transition{,1..2,7} (4 alike) : RateTransition  OutPortSampleTime=Ts_Control
  Rate Transition11 : RateTransition  OutPortSampleTime=Ts_Power
  Rate Transition3 : RateTransition  OutPortSampleTime=Ts_Power
  Rate Transition4 : RateTransition  OutPortSampleTime=Ts_Power
  Reactive Power Regulator : Subsystem
      settings: PortSchema="{\"entries\":[{\"content\":{\"sides\":[{\"content\":{\"connectorIds\":[\"In1\",\"In2\"]},\"type\":\"ConnectorPlacement.EquallySpacedRectSide\",\"uuid\":\"eeeb811d-908b-486e-b0fa-0b5fd0d6695a\"},{\"content\":{\"connectorIds\":[\"Out1\"],\"side\":\"RIGHT\"},\"type\":\"ConnectorPlacement.EquallySpacedRectSide\",\"uuid\":\"28c9bf02-c5ab-433a-87a9-c17e67d0c029\"},{\"content\":{\"side\":\"TOP\"},\"type\":\"ConnectorPlacement.EquallySpacedRectSide\",\"uuid\":\"fdca837a-4079-4910-a6d7-edbb284eaa51\"},{\"content\":{\"connectorIds\":[\"In3\",\"In4\"],\"side\":\"BOTTOM\"},\"type\":\"ConnectorPlacement.EquallySpacedRectSide\",\"uuid\":\"d2fa5805-110b-4a78-bf6e-301fd334a724\"}]},\"type\":\"ConnectorPlacement.EquallySpacedConnector\",\"uuid\":\"cbc8ea8f-55f5-4ff6-b34f-d5812b415dcf\"}],\"packageUris\":[\"http://schema.mathworks.com/mf0/Connector/R2020b\"],\"version\":\"1.0\"}"
  Switch : Switch  Criteria=u2 ~= 0  SaturateOnIntegerOverflow=off  InputSameDT=off
  Uref : Outport
  Meas : Outport  Port=2
  m1_dq : Outport  Port=3
  wt : Outport  Port=4
  wires:
  Mux1/1 -> Bus Creator/7  "PrefPmeas"
  "PLL, Measurements and Transformation"/4(P) -> Mux1/2, Active Power Regulator (Preg)/1(Pmeas)
  DC Voltage Regulator (VDCreg)/1(Id_ref) -> Mux/1
  "PLL, Measurements and Transformation"/2(wt) -> Rate Transition4/1, Current Regulator (Ireg)/4(wt)
  Demux1/1 -> Bus Creator/3  "Id"
  Vsec/1 -> Rate Transition1/1
  "PLL, Measurements and Transformation"/6(VdVq) -> Reactive Power Regulator/4(VdVq_mes), Current Regulator (Ireg)/2(VdVq)
  Mux2/1 -> [QrefQmeas]
  Rate Transition11/1 -> Uref/1
  "PLL, Measurements and Transformation"/5(Q) -> Mux2/2, Reactive Power Regulator/3(Qmes)
  [Pref] -> Active Power Regulator (Preg)/2(Pref), Mux1/1
  Isec/1 -> Rate Transition2/1
  [PQreg_On] -> Active Power Regulator (Preg)/3(On)
  [QrefQmeas] -> Bus Creator/8  "QrefQmeas"
  Current Regulator (Ireg)/2(m) -> Rate Transition3/1, Rate Transition7/1
  Demux3/2 -> Bus Creator/2  "Iqref"
  Rate Transition7/1 -> Bus Creator/5  "m"
  [Vdc_ref_Preg] -> Switch/1
  Demux3/1 -> Bus Creator/1  "Idref"
  Mux/1 -> Demux3/1, Current Regulator (Ireg)/1(IdIq_ref)
  Switch/1 -> DC Voltage Regulator (VDCreg)/1(Vdc_ref)
  Current Regulator (Ireg)/3(PIdq) -> Bus Creator/6  "PIdq"
  [Vdc1] -> Rate Transition/1
  PQreg_ON/1 -> Reactive Power Regulator/1(On), Switch/2
  Rate Transition1/1 -> "PLL, Measurements and Transformation"/1(Vabc)
  "PLL, Measurements and Transformation"/1(Freq) -> Current Regulator (Ireg)/3(Freq)
  Vdc_ref/1 -> Switch/3
  Active Power Regulator (Preg)/1(Vdc_ref) -> [Vdc_ref_Preg]
  Rate Transition2/1 -> "PLL, Measurements and Transformation"/2(Iabc)
  Rate Transition/1 -> DC Voltage Regulator (VDCreg)/3(Vdc_meas), Current Regulator (Ireg)/6(Vdc)
  [VDCreg_On] -> DC Voltage Regulator (VDCreg)/2(On)
  Demux1/2 -> Bus Creator/4  "Iq"
  "PLL, Measurements and Transformation"/3(IdIq) -> Current Regulator (Ireg)/5(IdIq), Demux1/1
  Qref/1 -> Mux2/1, Reactive Power Regulator/2(Qref)
  Current Regulator (Ireg)/1(Uref_ABC) -> Rate Transition11/1
  Bus Creator/1 -> Meas/1
  Reactive Power Regulator/1(Iq_ref) -> Mux/2
  Rate Transition3/1 -> m1_dq/1
  Rate Transition4/1 -> wt/1

== system x20240109_HVDCMMCInterconnection/Conv 2 ==
  On : Inport
  Add : Sum
  Constant : Constant  Value=0
  Constant2 : Constant  Value=Vnom_dc/2  SampleTime=Ts_Power
  Controlled Voltage Source : spsControlledVoltageSourceLib/Controlled Voltage Source  Initialize=off  Source_Type=AC  Amplitude=0  Phase=0  Frequency=0  Measurements=None
  Controlled Voltage Source1 : spsControlledVoltageSourceLib/Controlled Voltage Source  Initialize=off  Source_Type=AC  Amplitude=0  Phase=0  Frequency=0  Measurements=None
  Current Measurement1 : spsCurrentMeasurementLib/Current Measurement  PhasorSimulation=off  OutputType=Complex  PSBequivalent=0
  Current Measurement2 : spsCurrentMeasurementLib/Current Measurement  PhasorSimulation=off  OutputType=Complex  PSBequivalent=0
  Gain : Gain  Gain=0.5
  Gain1 : Gain  Gain=-1
  Ground1 : spsGroundLib/Ground  LConnTagsString=a
  Ground2 : spsGroundLib/Ground  LConnTagsString=a
  Ideal Switch : spsIdealSwitchLib/Ideal Switch  Ron=0.001  Lon=0  IC=0  Rs=1e6  Cs=inf  Measurements=off
  Ideal Switch1 : spsIdealSwitchLib/Ideal Switch  Ron=0.001  Lon=0  IC=0  Rs=1e6  Cs=inf  Measurements=off
  Switch : Switch  Criteria=u2 > Threshold  SaturateOnIntegerOverflow=off  InputSameDT=off
  Voltage Measurement : spsVoltageMeasurementLib/Voltage Measurement  PhasorSimulation=off  OutputType=Complex  PSBequivalent=0
  Voltage Measurement1 : spsVoltageMeasurementLib/Voltage Measurement  PhasorSimulation=off  OutputType=Complex  PSBequivalent=0
  Voltage Measurement2 : spsVoltageMeasurementLib/Voltage Measurement  PhasorSimulation=off  OutputType=Complex  PSBequivalent=0
  + : PMIOPort  Side=Left
  -- : PMIOPort  Port=2  Side=Left
  tag scope: Idc2=global, Vdc2=global, Vdc2b=global, Vdc2t=global
  wires:
  On/1 -> Ideal Switch1/1, Ideal Switch/1, Switch/2
  Current Measurement1/1 -> Add/1
  Current Measurement2/1 -> Gain1/1
  Add/1 -> Gain/1
  Gain/1 -> [Idc2]
  Gain1/1 -> Add/2
  Constant2/1 -> Switch/1
  Switch/1 -> Controlled Voltage Source/1, Controlled Voltage Source1/1
  Constant/1 -> Switch/3
  Voltage Measurement/1 -> [Vdc2]
  Voltage Measurement1/1 -> [Vdc2t]
  Voltage Measurement2/1 -> [Vdc2b]
  connections:
  Ideal Switch/LConn1 -- Current Measurement1/RConn1
  Controlled Voltage Source1/LConn1 -- Ideal Switch1/RConn1
  Ideal Switch/RConn1 -- Controlled Voltage Source/RConn1
  Controlled Voltage Source1/RConn1 -- Controlled Voltage Source/LConn1 -- Ground1/LConn1
  Current Measurement1/LConn1 -- Voltage Measurement/LConn1 -- +/RConn1 -- Voltage Measurement1/LConn1
  --/RConn1 -- Current Measurement2/LConn1 -- Voltage Measurement/LConn2 -- Voltage Measurement2/LConn2
  Current Measurement2/RConn1 -- Ideal Switch1/LConn1
  Voltage Measurement1/LConn2 -- Voltage Measurement2/LConn1 -- Ground2/LConn1

== system x20240109_HVDCMMCInterconnection/DC & converter 2 ==
  Add : Sum
  Cinv : spsSeriesRLCBranchLib/Series RLC Branch  LConnTagsString=__new0  RConnTagsString=__new0  BranchType=RC  Resistance=1e-3  Inductance=1e-3  SetiL0=off  InitialCurrent=0  Capacitance=C_PM/Nb_PM*3  Setx0=off  InitialVoltage=Vnom_dc/2  Measurements=None
  Cinv1 : spsSeriesRLCBranchLib/Series RLC Branch  LConnTagsString=__new0  RConnTagsString=__new0  BranchType=RC  Resistance=1e-3  Inductance=1e-3  SetiL0=off  InitialCurrent=0  Capacitance=C_PM/Nb_PM*3  Setx0=off  InitialVoltage=Vnom_dc/2  Measurements=None
  CnDC : spsSeriesRLCBranchLib/Series RLC Branch  LConnTagsString=__new0  RConnTagsString=__new0  BranchType=RC  Resistance=Rg  Inductance=1e-3  SetiL0=off  InitialCurrent=0  Capacitance=Cg  Setx0=off  InitialVoltage=Vnom_dc/2  Measurements=None
  CpDC : spsSeriesRLCBranchLib/Series RLC Branch  LConnTagsString=__new0  RConnTagsString=__new0  BranchType=RC  Resistance=Rg  Inductance=1e-3  SetiL0=off  InitialCurrent=0  Capacitance=Cg  Setx0=off  InitialVoltage=Vnom_dc/2  Measurements=None
  Gain : Gain  Gain=-0.5
  Gain1 : Gain  Gain=-1
  Ground2 : spsGroundLib/Ground  LConnTagsString=a
  Ground4 : spsGroundLib/Ground  LConnTagsString=a
  Idc1n : spsCurrentMeasurementLib/Current Measurement  PhasorSimulation=off  OutputType=Complex  PSBequivalent=0
  Idc1p : spsCurrentMeasurementLib/Current Measurement  PhasorSimulation=off  OutputType=Complex  PSBequivalent=0
  Vdc1 : spsVoltageMeasurementLib/Voltage Measurement  PhasorSimulation=off  OutputType=Complex  PSBequivalent=0
  Zcable1_1 : spsSeriesRLCBranchLib/Series RLC Branch  LConnTagsString=__new0  RConnTagsString=__new0  BranchType=RL  Resistance=R_cable  Inductance=L_cable  SetiL0=off  InitialCurrent=0  Capacitance=1e-6  Setx0=off  InitialVoltage=0  Measurements=None
  Zcable2_1 : spsSeriesRLCBranchLib/Series RLC Branch  LConnTagsString=__new0  RConnTagsString=__new0  BranchType=RL  Resistance=R_cable  Inductance=L_cable  SetiL0=off  InitialCurrent=0  Capacitance=1e-6  Setx0=off  InitialVoltage=0  Measurements=None
  Zcable5 : spsSeriesRLCBranchLib/Series RLC Branch  LConnTagsString=__new0  RConnTagsString=__new0  BranchType=RL  Resistance=1e-2+1e-3  Inductance=1e-4  SetiL0=off  InitialCurrent=0  Capacitance=1e-6  Setx0=off  InitialVoltage=0  Measurements=None
  Zcable6 : spsSeriesRLCBranchLib/Series RLC Branch  LConnTagsString=__new0  RConnTagsString=__new0  BranchType=RL  Resistance=1e-2+1e-3  Inductance=1e-4  SetiL0=off  InitialCurrent=0  Capacitance=1e-6  Setx0=off  InitialVoltage=0  Measurements=None
  1 : PMIOPort  Side=Left
  2 : PMIOPort  Port=2  Side=Left
  3 : PMIOPort  Port=3  Side=Right
  4 : PMIOPort  Port=4  Side=Right
  tag scope: Idc1=global, Vdc1=global
  wires:
  Vdc1/1 -> [Vdc1]
  Idc1p/1 -> Add/1
  Idc1n/1 -> Gain1/1
  Add/1 -> Gain/1
  Gain/1 -> [Idc1]
  Gain1/1 -> Add/2
  connections:
  Cinv1/LConn1 -- Ground2/LConn1 -- Cinv/RConn1
  Ground4/LConn1 -- CnDC/LConn1 -- CpDC/RConn1
  Zcable2_1/RConn1 -- CnDC/RConn1 -- Vdc1/LConn2 -- Idc1n/RConn1
  Zcable1_1/RConn1 -- Vdc1/LConn1 -- Idc1p/RConn1 -- CpDC/LConn1
  1/RConn1 -- Idc1p/LConn1
  Zcable6/RConn1 -- Zcable2_1/LConn1 -- Cinv1/RConn1
  Zcable5/LConn1 -- Zcable1_1/LConn1 -- Cinv/LConn1
  Idc1n/LConn1 -- 2/RConn1
  3/RConn1 -- Zcable5/RConn1
  4/RConn1 -- Zcable6/LConn1

== system x20240109_HVDCMMCInterconnection/Delay1 ==
  In1 : Inport
  Gain3 : Gain  Gain=0.5
  Sum4 : Sum  InputSameDT=on  SaturateOnIntegerOverflow=on  OutDataTypeStr=Inherit: Same as first input
  Unit Delay6 : UnitDelay  SampleTime=Ts_Power  HasFrameUpgradeWarning=on
  Out1 : Outport
  wires:
  In1/1 -> Sum4/2, Unit Delay6/1
  Unit Delay6/1 -> Sum4/1
  Sum4/1 -> Gain3/1
  Gain3/1 -> Out1/1

== system x20240109_HVDCMMCInterconnection/Delay5 ==
  In1 : Inport
  Gain3 : Gain  Gain=0.5
  Sum4 : Sum  InputSameDT=on  SaturateOnIntegerOverflow=on  OutDataTypeStr=Inherit: Same as first input
  Unit Delay6 : UnitDelay  SampleTime=Ts_Power  HasFrameUpgradeWarning=on
  Out1 : Outport
  wires:
  In1/1 -> Sum4/2, Unit Delay6/1
  Unit Delay6/1 -> Sum4/1
  Sum4/1 -> Gain3/1
  Gain3/1 -> Out1/1

== system x20240109_HVDCMMCInterconnection/Delay6 ==
  In1 : Inport
  Gain3 : Gain  Gain=0.5
  Sum4 : Sum  InputSameDT=on  SaturateOnIntegerOverflow=on  OutDataTypeStr=Inherit: Same as first input
  Unit Delay6 : UnitDelay  SampleTime=Ts_Power  HasFrameUpgradeWarning=on
  Out1 : Outport
  wires:
  In1/1 -> Sum4/2, Unit Delay6/1
  Unit Delay6/1 -> Sum4/1
  Sum4/1 -> Gain3/1
  Gain3/1 -> Out1/1

== system x20240109_HVDCMMCInterconnection/Delay7 ==
  In1 : Inport
  Gain3 : Gain  Gain=0.5
  Sum4 : Sum  InputSameDT=on  SaturateOnIntegerOverflow=on  OutDataTypeStr=Inherit: Same as first input
  Unit Delay6 : UnitDelay  SampleTime=Ts_Power  HasFrameUpgradeWarning=on
  Out1 : Outport
  wires:
  In1/1 -> Sum4/2, Unit Delay6/1
  Unit Delay6/1 -> Sum4/1
  Sum4/1 -> Gain3/1
  Gain3/1 -> Out1/1

== system x20240109_HVDCMMCInterconnection/Delay8 ==
  In1 : Inport
  Gain3 : Gain  Gain=0.5
  Sum4 : Sum  InputSameDT=on  SaturateOnIntegerOverflow=on  OutDataTypeStr=Inherit: Same as first input
  Unit Delay6 : UnitDelay  SampleTime=Ts_Power  HasFrameUpgradeWarning=on
  Out1 : Outport
  wires:
  In1/1 -> Sum4/2, Unit Delay6/1
  Unit Delay6/1 -> Sum4/1
  Sum4/1 -> Gain3/1
  Gain3/1 -> Out1/1

== system x20240109_HVDCMMCInterconnection/Delay9 ==
  In1 : Inport
  Gain3 : Gain  Gain=0.5
  Sum4 : Sum  InputSameDT=on  SaturateOnIntegerOverflow=on  OutDataTypeStr=Inherit: Same as first input
  Unit Delay6 : UnitDelay  SampleTime=Ts_Power  HasFrameUpgradeWarning=on
  Out1 : Outport
  wires:
  In1/1 -> Sum4/2, Unit Delay6/1
  Unit Delay6/1 -> Sum4/1
  Sum4/1 -> Gain3/1
  Gain3/1 -> Out1/1

== system x20240109_HVDCMMCInterconnection/Discrete State-Space1 ==
  note: Implement discretized state-space model using Tustin or TBE method
      |
      | BE      -> SM.DSSmethod=1
      | Tustin  -> SM.DSSmethod=2
      |
      |
      | Tustin
      | ------
      | Ad = inv(I - Ts/2*A)*(I + Ts/2*A)
      | Bd = inv(I - Ts/2*A)*B
      | Cd = C*inv(I - Ts/2*A)*Ts
      | Dd = C*inv(I - Ts/2*A)*B*Ts/2  + D  =  Cd*B/2
      |
      | TBE
      | ---
      | Ad = inv(I - Ts*A)
      | Bd = inv(I - Ts*A)*B
      | Cd = C*inv(I - Ts*A)*Ts
      | Dd = C*inv(I - Ts*A)*B*Ts  + D  =  Cd*B
      |
      | I = eye(SM.nState,SM.nState)
  U : Inport
  Constant : Constant  Value=Ad1
  Constant1 : Constant  Value=Cd1
  Constant2 : Constant  Value=Bd1
  Constant3 : Constant  Value=Dd1
  Constant5 : Constant  Commented=on  Value=sps_AC.A
  Constant6 : Constant  Commented=on  Value=sps_AC.B
  Constant7 : Constant  Commented=on  Value=sps_AC.C
  Constant8 : Constant  Commented=on  Value=sps_AC.D
  Discretize BE or Tustin : Subsystem  Commented=on  AncestorBlock="DQN_Machines/DQN_Mac_V1/Discretize  BE or Tustin"
  Ihistory_Flux : Subsystem  AncestorBlock=DQN_Machines/DQN_Mac_V1/Ihistory_Flux
  Y : Outport
  wires:
  Constant/1 -> [Ad]
  Constant2/1 -> [Bd]
  Constant1/1 -> [Cd]
  Constant3/1 -> [Dd1]
  Constant7/1 -> Discretize BE or Tustin/3(C)
  Constant6/1 -> Discretize BE or Tustin/2(B)
  Constant8/1 -> Discretize BE or Tustin/4(D)
  Constant5/1 -> Discretize BE or Tustin/1(A)
  U/1 -> Ihistory_Flux/1(u)
  Ihistory_Flux/1(Ihyst) -> Y/1
  [Ad] -> Ihistory_Flux/2(Ad)
  [Bd] -> Ihistory_Flux/3(Bd)
  [Cd] -> Ihistory_Flux/4(Cd)
  [Dd1] -> Ihistory_Flux/5(D)
